simulink library "ayazController_cl"  (R2018b)
settings: Solver=VariableStepAuto  StartTime=0.0  StopTime=10.0  RelTol=1e-3
undefined symbols (not defined in the file or in its folder): elevon_max_deflection, kd_aileron, kd_elev, Kd_p, Kd_r, Kd_z, ki_aileron, ki_elev, Ki_p, Ki_r, kp_aileron, kp_elev, Kp_p, Kp_r, Kp_z, P_cs_mat, P_inv, t_aileron, t_elev, wce_p, wce_r, wce_z, winc_vel_up_lims
settings Model: Creator=mcobb  LastModifiedBy=embeato2

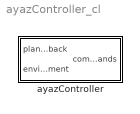
== system ayazController_cl ==
  ayazController : Subsystem  VariantControl=VSS_controller_ayazController

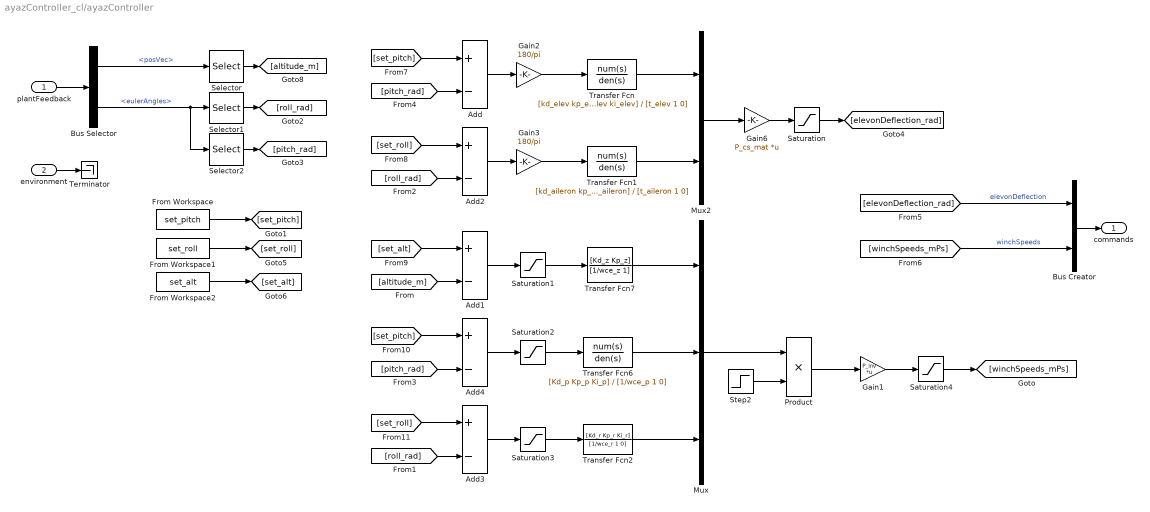
== system ayazController_cl/ayazController ==
  plantFeedback : Inport  OutDataTypeStr=Bus: plantBus
  environment : Inport  Port=2  OutDataTypeStr=Bus: envBus
  Add{,1..4} (5 alike) : Sum  Inputs=+-
  Bus Creator : BusCreator  Inputs=2
  Bus Selector : BusSelector  OutputSignals=posVec,eulerAngles
  From Workspace : FromWorkspace  VariableName=set_pitch  SampleTime=0
  From Workspace1 : FromWorkspace  VariableName=set_roll  SampleTime=0
  From Workspace2 : FromWorkspace  VariableName=set_alt  SampleTime=0
  Gain1 : Gain  Gain=P_inv  Multiplication=Matrix(K*u)
  Gain2 : Gain  Gain=180/pi
  Gain3 : Gain  Gain=180/pi
  Gain6 : Gain  Gain=P_cs_mat  Multiplication=Matrix(K*u)
  Mux : Mux  Inputs=3
  Mux2 : Mux  Inputs=2
  Product : Product
  Saturation : Saturate  UpperLimit=elevon_max_deflection  LowerLimit=-elevon_max_deflection
  Saturation1 : Saturate  UpperLimit=5  LowerLimit=-5
  Saturation2 : Saturate  UpperLimit=5  LowerLimit=-5
  Saturation3 : Saturate  UpperLimit=5  LowerLimit=-5
  Saturation4 : Saturate  UpperLimit=winc_vel_up_lims  LowerLimit=-winc_vel_up_lims
  Selector : Selector  InputPortWidth=3  IndexOptions=Index vector (dialog)  Indices=3  OutputSizes=1
  Selector1 : Selector  InputPortWidth=3  IndexOptions=Index vector (dialog)  Indices=1  OutputSizes=1
  Selector2 : Selector  InputPortWidth=3  IndexOptions=Index vector (dialog)  Indices=2  OutputSizes=1
  Step2 : Step  Time=0  SampleTime=0
  Terminator : Terminator
  Transfer Fcn : TransferFcn  Numerator=[kd_elev kp_elev ki_elev]  Denominator=[t_elev 1 0]
  Transfer Fcn1 : TransferFcn  Numerator=[kd_aileron kp_aileron ki_aileron]  Denominator=[t_aileron 1 0]
  Transfer Fcn2 : TransferFcn  Numerator=[Kd_r Kp_r Ki_r]  Denominator=[1/wce_r 1 0]
  Transfer Fcn6 : TransferFcn  Numerator=[Kd_p Kp_p Ki_p]  Denominator=[1/wce_p 1 0]
  Transfer Fcn7 : TransferFcn  Numerator=[Kd_z Kp_z]  Denominator=[1/wce_z 1]
  commands : Outport  OutDataTypeStr=Bus: ctrlBus
  wires:
  Product/1 -> Gain1/1
  Mux2/1 -> Gain6/1
  Transfer Fcn1/1 -> Mux2/2
  Transfer Fcn/1 -> Mux2/1
  [roll_rad] -> Add2/2
  Add2/1 -> Gain3/1
  [pitch_rad] -> Add/2
  Gain6/1 -> Saturation/1
  Gain2/1 -> Transfer Fcn/1
  Gain3/1 -> Transfer Fcn1/1
  Add/1 -> Gain2/1
  Step2/1 -> Product/2
  Mux/1 -> Product/1
  Gain1/1 -> Saturation4/1
  Saturation2/1 -> Transfer Fcn6/1
  Saturation3/1 -> Transfer Fcn2/1
  Saturation1/1 -> Transfer Fcn7/1
  [pitch_rad] -> Add4/2
  [roll_rad] -> Add3/2
  Transfer Fcn2/1 -> Mux/3
  Add4/1 -> Saturation2/1
  [altitude_m] -> Add1/2
  Add1/1 -> Saturation1/1
  Transfer Fcn6/1 -> Mux/2
  Transfer Fcn7/1 -> Mux/1
  Add3/1 -> Saturation3/1
  Selector/1 -> [altitude_m]
  Selector1/1 -> [roll_rad]
  Bus Selector/2 -> Selector2/1, Selector1/1  "<eulerAngles>"
  environment/1 -> Terminator/1
  plantFeedback/1 -> Bus Selector/1
  Bus Selector/1 -> Selector/1  "<posVec>"
  Selector2/1 -> [pitch_rad]
  [winchSpeeds_mPs] -> Bus Creator/2  "winchSpeeds"
  [elevonDeflection_rad] -> Bus Creator/1  "elevonDeflection"
  Bus Creator/1 -> commands/1
  Saturation4/1 -> [winchSpeeds_mPs]
  Saturation/1 -> [elevonDeflection_rad]
  From Workspace/1 -> [set_pitch]
  From Workspace1/1 -> [set_roll]
  From Workspace2/1 -> [set_alt]
  [set_pitch] -> Add/1
  [set_alt] -> Add1/1
  [set_pitch] -> Add4/1
  [set_roll] -> Add3/1
  [set_roll] -> Add2/1
